simulink library "INT_RailP_VD"  (R2016b)
settings: Solver=VariableStepAuto  StartTime=0.0  StopTime=10.0  RelTol=1e-3
settings Model: Creator=liutao  LastModifiedBy=liutao

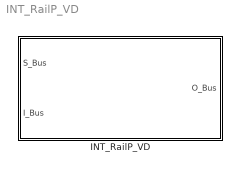
== system INT_RailP_VD ==
  INT_RailP_VD : Subsystem

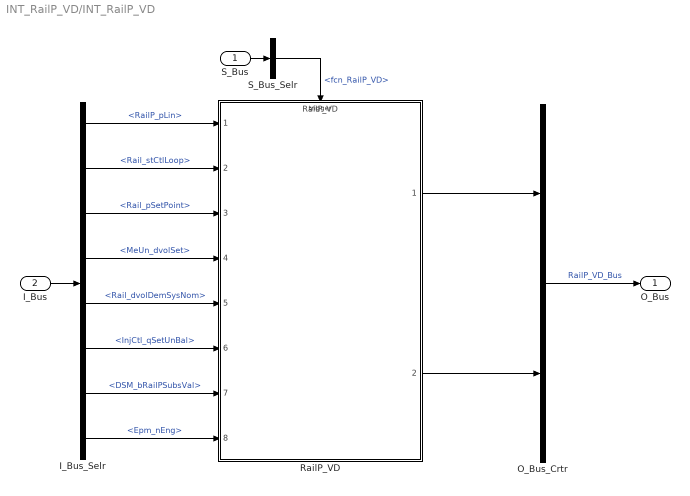
== system INT_RailP_VD/INT_RailP_VD ==
  S_Bus : Inport
  I_Bus : Inport  Port=2
  I_Bus_Selr : BusSelector  OutputSignals=RailP_pLin,Rail_stCtlLoop,Rail_pSetPoint,MeUn_dvolSet,Rail_dvolDemSysNom,InjCtl_qSetUnBal,DSM_bRailPSubsVal,Epm_nEng
  O_Bus_Crtr : BusCreator  Inputs=2
  RailP_VD : ModelReference  ModelNameDialog=RailP_VD  SimulationMode=Normal  ModelReferenceVersion=1.40  TriggerPortName=function  TriggerPortTriggerType=function-call  TriggerPortStatesWhenEnabling=held
  S_Bus_Selr : BusSelector  OutputSignals=fcn_RailP_VD
  O_Bus : Outport
  wires:
  S_Bus_Selr/1 -> RailP_VD/Trigger  "<fcn_RailP_VD>"
  S_Bus/1 -> S_Bus_Selr/1
  I_Bus/1 -> I_Bus_Selr/1
  I_Bus_Selr/1 -> RailP_VD/1  "<RailP_pLin>"
  I_Bus_Selr/2 -> RailP_VD/2  "<Rail_stCtlLoop>"
  I_Bus_Selr/3 -> RailP_VD/3  "<Rail_pSetPoint>"
  I_Bus_Selr/4 -> RailP_VD/4  "<MeUn_dvolSet>"
  I_Bus_Selr/5 -> RailP_VD/5  "<Rail_dvolDemSysNom>"
  I_Bus_Selr/6 -> RailP_VD/6  "<InjCtl_qSetUnBal>"
  I_Bus_Selr/7 -> RailP_VD/7  "<DSM_bRailPSubsVal>"
  I_Bus_Selr/8 -> RailP_VD/8  "<Epm_nEng>"
  O_Bus_Crtr/1 -> O_Bus/1  "RailP_VD_Bus"
  RailP_VD/1 -> O_Bus_Crtr/1
  RailP_VD/2 -> O_Bus_Crtr/2
